simulink library "VariousBlocksLibrary"  (R2015b)
settings: Solver=ode45  StartTime=0.0  StopTime=10.0  RelTol=1e-3
undefined symbols (not defined in the file or in its folder): LopesParams
undefined symbols (not defined in the file): LopesParamsSendDataArrayLen
libraries: simulink x17, dspmtrx3 x9, LopesDevelopmentLibrary x2, LopesLibrary x1, VariousBlocksLibrary x1
(part 1 of 2)
settings Model: xpc_rtwmakecfg_data=_xpcnblib__xpciplib__xpcetherlib__xpcether8255xlib__xpcetherGbElib_  Creator=Administrator  LastModifiedBy=symbitron
settings DataIOCC: SaveFormat=Array  SignalLoggingSaveFormat=ModelDataLogs
settings OptimizationCC: ExpressionDepthLimit=2147483647
settings DebuggingCC: UnderspecifiedInitializationDetection=Classic  MergeDetectMultiDrivingBlocksExec=none  SolverPrmCheckMsg=warning  FcnCallInpInsideContextMsg=UseLocalSettings  StateNameClashWarn=warning
settings HardwareCC: ProdBitPerPointer=32  ProdLargestAtomicFloat=None  ProdIntDivRoundTo=Undefined  ProdEndianess=Unspecified  ProdWordSize=32  ProdHWDeviceType=32-bit Generic
settings GRTTargetCC: GeneratePreprocessorConditionals=Disable all  CombineOutputUpdateFcns=off  GRTInterface=on
settings ConfigComp: CovModelRefEnable=Off

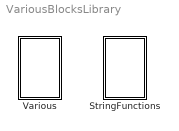
== system VariousBlocksLibrary ==
  StringFunctions : Subsystem
  Various : Subsystem

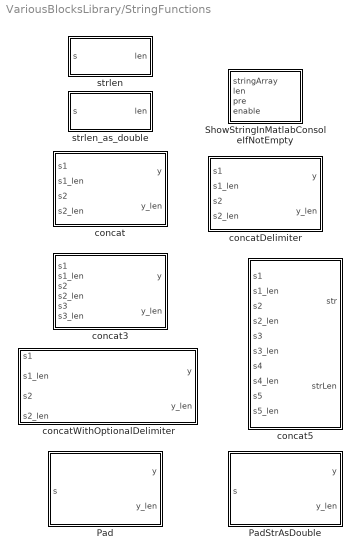
== system VariousBlocksLibrary/StringFunctions ==
  Pad : Subsystem  mask{outArrayLen=100}
      mask prompts: outArrayLen "Size of output array"
  PadStrAsDouble : Subsystem  mask{outArrayLen=LopesParams.exceptionStrArrayLen}
      mask prompts: outArrayLen "Size of output array"
  ShowStringInMatlabConsoleIfNotEmpty : MATLAB Function  TreatAsAtomicUnit=on
  concat : MATLAB Function  TreatAsAtomicUnit=on
  concat3 : MATLAB Function  TreatAsAtomicUnit=on
  concat5 : Subsystem  mask{outStrLen=LopesParamsSendDataArrayLen}
      mask prompts: outStrLen "Length of output array"
  concatDelimiter : MATLAB Function  TreatAsAtomicUnit=on
  concatWithOptionalDelimiter : MATLAB Function  TreatAsAtomicUnit=on
  strlen : MATLAB Function  TreatAsAtomicUnit=on
  strlen_as_double : MATLAB Function  TreatAsAtomicUnit=on

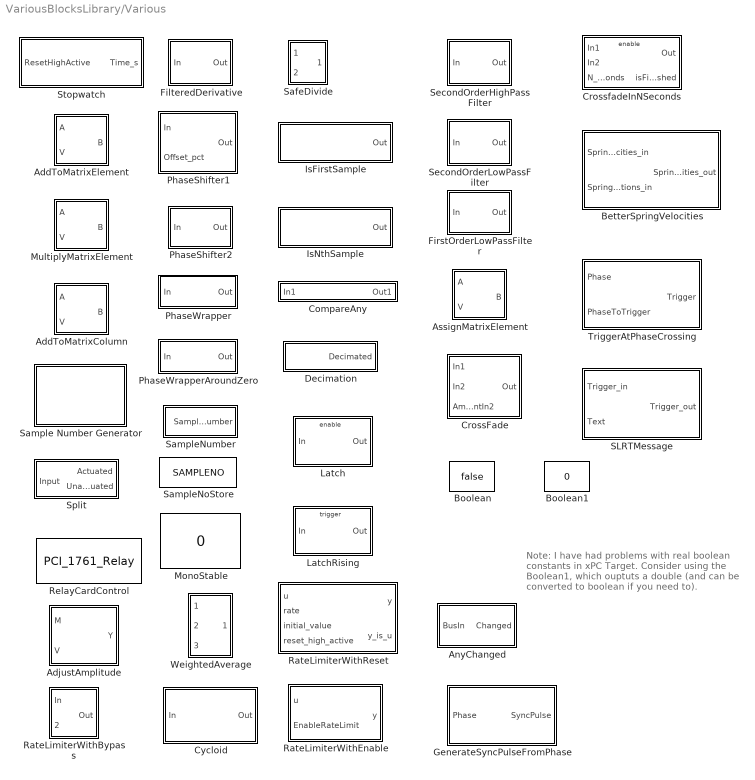
== system VariousBlocksLibrary/Various ==
  note: Note: I have had problems
      | with real boolean constants
      | in xPC Target. Consider
      | using the Boolean1, which ouptuts
      | a double (and can be converted to boolean
      | if you need to).
  AddToMatrixColumn : Subsystem  mask{col=1, minimum=-inf, maximum=inf}
      mask prompts: col "Column (1-based)"
      mask Display:
      | plot([15,10,10,15],[0,0,75,75])
      | plot([70,75,75,70],[0,0,75,75])
      | plot(0,-5)
      | plot(85,85)
      | plot([55,55],[60,70])
      | plot([50,60],[65,65])
      | plot([55,55],[35,45])
      | plot([50,60],[40,40])
      | plot([55,55],[10,20])
      | plot([50,60],[15,15])
  AddToMatrixElement : Subsystem  mask{row=1, col=1, minimum=-inf, maximum=inf}
      mask prompts: row "Row (1-based)"; col "Column (1-based)"
      mask Display:
      | plot([15,10,10,15],[0,0,75,75])
      | plot([70,75,75,70],[0,0,75,75])
      | plot(0,-5)
      | plot(85,85)
      | plot([55,55],[70,60])
      | plot([50,60],[65,65])
  AdjustAmplitude : Subsystem
  AnyChanged : Subsystem
  AssignMatrixElement : Subsystem  mask{row=3, col=2, minimum=-inf, maximum=inf}
      mask prompts: row "Row (1-based)"; col "Column (1-based)"; minimum "Minimum value"; maximum "Maximum value"
      mask Display:
      | plot([15,10,10,15],[0,0,75,75])
      | plot([70,75,75,70],[0,0,75,75])
      | plot(0,-5)
      | plot(85,85)
      | plot([50,60,60,50,50],[60,60,70,70,60])
  BetterSpringVelocities : Subsystem
  Boolean : Constant  Value=false  OutDataTypeStr=boolean
      settings: OpenFcn=|
      | b = get_param(gcb,'value');
      | if (strcmp(b,'true')),
      |   set_param (gcb,'value','false');
      | else
      |   set_param(gcb,'value','true');
      | end;
  Boolean1 : Constant  Value=0  OutDataTypeStr=double
      settings: OpenFcn=|
      | b = get_param(gcb,'value');
      | if (strcmp(b,'1')),
      |   set_param (gcb,'value','0');
      | else
      |   set_param(gcb,'value','1');
      | end;
  CompareAny : Subsystem  mask{values=[3,4]}
      mask Display: disp(['==(',num2strjoin(values,'||'),')'])
  CrossFade : Subsystem
  CrossfadeInNSeconds : Subsystem
  Cycloid : Subsystem
  Decimation : Subsystem  mask{Decimation=1}
      mask prompts: Decimation "Decimation Amount"
      mask TypeOptions Decimation: DecimationAmount/Value
      mask Display: disp(['Decimation: ',num2str(eval(get_param([gcb,'/DecimationAmount'],'Value')))])
  FilteredDerivative : Subsystem  mask{w=10*(2*pi), z=0.7}
      mask prompts: w "Cut off omega [rad/s]"; z "Zeta"
  FirstOrderLowPassFilter : Subsystem  mask{Tau=1}
  GenerateSyncPulseFromPhase : Subsystem
  IsFirstSample : Subsystem  InitFcn=|
      | return; %Disable this becasue it doesnt work!                                                                                                                                                          
      | h = gcb;                                                                                                                                                                                               
      | n = 0; % Number of enable blocks detected upstream                                                                                                                                                     
      | t = []; % type of enable blocks                                                                                                                                                                        
      | while 1,                                                                                                                                                                                               
      |   % Find parent                                                                                                                                                                                        
      |   h = get_param(h,'parent');                                                                                                                                                                           
      |   if (strcmp(h,'')),                                                                                                                                                                                   
      |       % Then we've reached the root                                                                                                                                                                    
      |       break;                                                                                                                                                                                           
      |   end;                                                                                                                                                                                                 
      |   % and check if it has an enable port                                                                                                                                                                 
      |   e = find_system(h,'searchdepth',1, 'BlockType','EnablePort');                                                                                                                                        
      |   if (numel(e)==1),                                                                                                                                                                                    
      |     s = get_param(e{1},'StatesWhenEnabling');                                                                                                                                                          
      |     n=n+1;                                                                                                                                                                                             
      |     if (strcmp(s,'held')),                                                                                                                                                                             
      |         t=[t;'h']; %#ok<AGROW>                                                                                                                                                                         
      |     else                                                                                                                                                                                               
      |         t=[t;'r']; %#ok<AGROW>                                                                                                                                                                         
      |     end;                                                                                                                                                                                               
      |   elseif (numel(e)>1),                                                                                                                                                                                 
      |       error('hun? Multiple enable blocks!')                                                                                                                                                            
      |   end;                                                                                                                                                                                                 
      | end;                                                                                                                                                                                                   
      |                                                                                                                                                                                                        
      | if (n==0),                                                                                                                                                                                             
      |     warning('Warning: %s - The block is not inside an enabled block',gcb)                                                                                                                              
      | elseif (n==1),                                                                                                                                                                                         
      |     if (t(1)=='r')                                                                                                                                                                                     
      |         % This is okay, do nothing                                                                                                                                                                     
      |     else                                                                                                                                                                                               
      |         warning('Warning: %s - This block is inside an enabled block which has its "State when enabling" set to "held". Usually you want it set to "reset" for correct operation.',gcb);               
      |     end;                                                                                                                                                                                               
      | else % n>1                                                                                                                                                                                             
      |     warning('Warning: %s - This block is inside multiple nested enabled blocks. Check which blocks are "held" and which are "reset". You usually want to have at least one "reset" enabled block',gcb);
      | end;
  IsNthSample : Subsystem  InitFcn=|  mask{N=40}
      | return; %Disable this becasue it doesnt work!                                                                                                                                                          
      | h = gcb;                                                                                                                                                                                               
      | n = 0; % Number of enable blocks detected upstream                                                                                                                                                     
      | t = []; % type of enable blocks                                                                                                                                                                        
      | while 1,                                                                                                                                                                                               
      |   % Find parent                                                                                                                                                                                        
      |   h = get_param(h,'parent');                                                                                                                                                                           
      |   if (strcmp(h,'')),                                                                                                                                                                                   
      |       % Then we've reached the root                                                                                                                                                                    
      |       break;                                                                                                                                                                                           
      |   end;                                                                                                                                                                                                 
      |   % and check if it has an enable port                                                                                                                                                                 
      |   e = find_system(h,'searchdepth',1, 'BlockType','EnablePort');                                                                                                                                        
      |   if (numel(e)==1),                                                                                                                                                                                    
      |     s = get_param(e{1},'StatesWhenEnabling');                                                                                                                                                          
      |     n=n+1;                                                                                                                                                                                             
      |     if (strcmp(s,'held')),                                                                                                                                                                             
      |         t=[t;'h']; %#ok<AGROW>                                                                                                                                                                         
      |     else                                                                                                                                                                                               
      |         t=[t;'r']; %#ok<AGROW>                                                                                                                                                                         
      |     end;                                                                                                                                                                                               
      |   elseif (numel(e)>1),                                                                                                                                                                                 
      |       error('hun? Multiple enable blocks!')                                                                                                                                                            
      |   end;                                                                                                                                                                                                 
      | end;                                                                                                                                                                                                   
      |                                                                                                                                                                                                        
      | if (n==0),                                                                                                                                                                                             
      |     warning('Warning: %s - The block is not inside an enabled block',gcb)                                                                                                                              
      | elseif (n==1),                                                                                                                                                                                         
      |     if (t(1)=='r')                                                                                                                                                                                     
      |         % This is okay, do nothing                                                                                                                                                                     
      |     else                                                                                                                                                                                               
      |         warning('Warning: %s - This block is inside an enabled block which has its "State when enabling" set to "held". Usually you want it set to "reset" for correct operation.',gcb);               
      |     end;                                                                                                                                                                                               
      | else % n>1                                                                                                                                                                                             
      |     warning('Warning: %s - This block is inside multiple nested enabled blocks. Check which blocks are "held" and which are "reset". You usually want to have at least one "reset" enabled block',gcb);
      | end;
  Latch : Subsystem  mask{ic=0}
      mask prompts: ic "Initial Condition"
  LatchRising : Subsystem  mask{ic=0}
      mask prompts: ic "Initial Condition"
  MonoStable : Constant  Value=0
      settings: OpenFcn=set_param(gcb,'Value','1');tname = ['toggletimer_' gcb];delete(timerfind('name',tname));t = timer('timerfcn', ['set_param(''',gcb,''',''Value'',''0'')'],'executionmode','singleshot','startdelay',1,'name',tname);start(t);
      mask Display: fprintf('PushToTrigger\n%s',get_param(gcb,'value'))
  MultiplyMatrixElement : Subsystem  mask{row=1, col=1, minimum=-inf, maximum=inf}
      mask prompts: row "Row (1-based)"; col "Column (1-based)"; minimum "Minimum value"; maximum "Maximum value"
      mask Display:
      | plot([15,10,10,15],[0,0,75,75])
      | plot([70,75,75,70],[0,0,75,75])
      | plot(0,-5)
      | plot(85,85)
      | plot([50,60],[70,60])
      | plot([50,60],[60,70])
  PhaseShifter1 : Subsystem
  PhaseShifter2 : Subsystem
  PhaseWrapper : Subsystem
  PhaseWrapperAroundZero : Subsystem
  RateLimiterWithBypass : Subsystem  mask{up=3, down=-3}
      mask prompts: up "Rising slew rate:"; down "Falling slew rate:"
      mask help: If Bypass is nonzero, the rate-limiting functionality is bypassed, and the output is made equal to the input immediately.
  RateLimiterWithEnable : Subsystem  mask{RisingSlewRate=0.5, FallingSlewRate=-0.5}
      mask prompts: RisingSlewRate "Rising Slew Rate:"; FallingSlewRate "Falling Slew Rate:"
  RateLimiterWithReset : Subsystem
  RelayCardControl : S-Function  FunctionName=PCI_1761_Relay  Parameters=baseaddress  SFunctionDeploymentMode=off  EnableBusSupport=off  mask{baseaddress=hex2dec('e000')}
      mask prompts: baseaddress "PCI Base Address (e.g. 0x0300)"
  SLRTMessage : Subsystem
  SafeDivide : Subsystem
      mask Display:
      | port_label('input',1,'X')
      | port_label('input',2,'/')
      | port_label('output',1,'')
  Sample Number Generator : Subsystem
      mask Display: disp('Sample Number\nGenerator')
  SampleNoStore : DataStoreMemory  DataStoreName=SAMPLENO  ReadBeforeWriteMsg=warning  WriteAfterWriteMsg=warning  WriteAfterReadMsg=warning
  SampleNumber : Subsystem
  SecondOrderHighPassFilter : Subsystem  mask{w=10*(2*pi), z=0.7}
      mask prompts: w "Cut off omega [rad/s]"; z "Zeta"
  SecondOrderLowPassFilter : Subsystem  mask{w=10*(2*pi), z=0.7}
      mask prompts: w "Cut off omega [rad/s]"; z "Zeta"
  Split : Subsystem
  Stopwatch : Subsystem
  TriggerAtPhaseCrossing : Subsystem
  WeightedAverage : Subsystem

== system VariousBlocksLibrary/StringFunctions/Pad ==
  s : Inport
  pad : MATLAB Function  TreatAsAtomicUnit=on
  y : Outport
  y_len : Outport  Port=2
  wires:
  pad/1(y) -> y/1
  s/1 -> pad/1(s)
  pad/2(y_len) -> y_len/1

== system VariousBlocksLibrary/StringFunctions/PadStrAsDouble ==
  note: This block pads a string array; the output is as an array of doubles
      | (needed for exception blocks).
  s : Inport
  Data Type Conversion : DataTypeConversion  OutDataTypeStr=double
  pad : MATLAB Function  TreatAsAtomicUnit=on
  y : Outport
  y_len : Outport  Port=2
  wires:
  Data Type Conversion/1 -> y/1
  pad/1(y) -> Data Type Conversion/1
  s/1 -> pad/1(s)
  pad/2(y_len) -> y_len/1

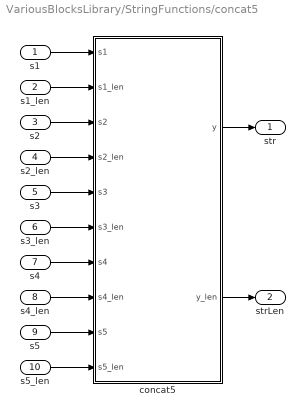
== system VariousBlocksLibrary/StringFunctions/concat5 ==
  s1 : Inport
  s1_len : Inport  Port=2
  s2 : Inport  Port=3
  s2_len : Inport  Port=4
  s3 : Inport  Port=5
  s3_len : Inport  Port=6
  s4 : Inport  Port=7
  s4_len : Inport  Port=8
  s5 : Inport  Port=9
  s5_len : Inport  Port=10
  concat5 : MATLAB Function  TreatAsAtomicUnit=on
  str : Outport
  strLen : Outport  Port=2
  wires:
  s5_len/1 -> concat5/10(s5_len)
  s3_len/1 -> concat5/6(s3_len)
  s3/1 -> concat5/5(s3)
  concat5/1(y) -> str/1
  s1_len/1 -> concat5/2(s1_len)
  s2/1 -> concat5/3(s2)
  s4/1 -> concat5/7(s4)
  s2_len/1 -> concat5/4(s2_len)
  s4_len/1 -> concat5/8(s4_len)
  s5/1 -> concat5/9(s5)
  s1/1 -> concat5/1(s1)
  concat5/2(y_len) -> strLen/1

== system VariousBlocksLibrary/Various/AddToMatrixColumn ==
  A : Inport
  V : Inport  Port=2
  Maximum : Constant  Value=maximum
  Minimum : Constant  Value=minimum
  Overwrite Values : dspmtrx3/Overwrite Values  OverWriteDiag=Submatrix  valFrom2ndIP=Second input port  ConstValue=0  RowSpan=All rows  RowStartMode=Index  RowStartIndex=row  RowEndMode=Last  RowEndIndex=1  ColSpan=One column  ColStartMode=Index  ColStartIndex=col  ColEndMode=Last  ColEndIndex=1  DiagSpan=Range of elements  DiagStartMode=Index  DiagStartIndex=2  DiagEndMode=Index  DiagEndIndex=4
  Saturation Dynamic : simulink/Discontinuities/Saturation Dynamic  OutMin=[]  OutMax=[]  OutDataTypeStr=Inherit: Same as second input  OutDataType=fixdt(1, 16)  OutScaling=2^-10  DoSatur=off
  Submatrix : dspmtrx3/Submatrix  RowSpan=All rows  RowStartMode=Index  RowStartIndex=row  RowEndMode=Index  RowEndIndex=1  ColSpan=One column  ColStartMode=Index  ColStartIndex=col  ColEndMode=Last  ColEndIndex=1
  Sum : Sum  Inputs=|++
  B : Outport
  wires:
  Minimum/1 -> Saturation Dynamic/3
  Maximum/1 -> Saturation Dynamic/1
  Saturation Dynamic/1 -> Overwrite Values/2
  Sum/1 -> Saturation Dynamic/2
  A/1 -> Submatrix/1, Overwrite Values/1
  Overwrite Values/1 -> B/1
  Submatrix/1 -> Sum/1
  V/1 -> Sum/2

== system VariousBlocksLibrary/Various/AddToMatrixElement ==
  A : Inport
  V : Inport  Port=2
  Maximum : Constant  Value=maximum
  Minimum : Constant  Value=minimum
  Overwrite Values : dspmtrx3/Overwrite Values  OverWriteDiag=Submatrix  valFrom2ndIP=Second input port  ConstValue=0  RowSpan=One row  RowStartMode=Index  RowStartIndex=row  RowEndMode=Last  RowEndIndex=1  ColSpan=One column  ColStartMode=Index  ColStartIndex=col  ColEndMode=Last  ColEndIndex=1  DiagSpan=Range of elements  DiagStartMode=Index  DiagStartIndex=2  DiagEndMode=Index  DiagEndIndex=4
  Saturation Dynamic : simulink/Discontinuities/Saturation Dynamic  OutMin=[]  OutMax=[]  OutDataTypeStr=Inherit: Same as second input  OutDataType=fixdt(1, 16)  OutScaling=2^-10  DoSatur=off
  Submatrix : dspmtrx3/Submatrix  RowSpan=One row  RowStartMode=Index  RowStartIndex=row  RowEndMode=Index  RowEndIndex=1  ColSpan=One column  ColStartMode=Index  ColStartIndex=col  ColEndMode=Last  ColEndIndex=1
  Sum : Sum  Inputs=|++
  B : Outport
  wires:
  V/1 -> Sum/2
  Submatrix/1 -> Sum/1
  Overwrite Values/1 -> B/1
  A/1 -> Overwrite Values/1, Submatrix/1
  Sum/1 -> Saturation Dynamic/2
  Saturation Dynamic/1 -> Overwrite Values/2
  Maximum/1 -> Saturation Dynamic/1
  Minimum/1 -> Saturation Dynamic/3

== system VariousBlocksLibrary/Various/AdjustAmplitude ==
  note: This block multiplies all positions, velocities and accelerations by input V;
      | in other words,  it just scales the amplitude of the total curve.
  M : Inport
  V : Inport  Port=2
  Matrix Concatenate : Concatenate  Mode=Multidimensional array  ConcatenateDimension=2
  Product : Product  RndMeth=Zero
  angle_vel_acc : dspmtrx3/Submatrix  RowSpan=All rows  RowStartMode=First  RowStartIndex=1  RowEndMode=Last  RowEndIndex=1  ColSpan=Range of columns  ColStartMode=Index  ColStartIndex=2  ColEndMode=Last  ColEndIndex=1
  times : dspmtrx3/Submatrix  RowSpan=All rows  RowStartMode=First  RowStartIndex=1  RowEndMode=Last  RowEndIndex=1  ColSpan=One column  ColStartMode=First  ColStartIndex=1  ColEndMode=Last  ColEndIndex=1
  Y : Outport
  wires:
  Product/1 -> Matrix Concatenate/2
  times/1 -> Matrix Concatenate/1
  angle_vel_acc/1 -> Product/1
  Matrix Concatenate/1 -> Y/1
  M/1 -> times/1, angle_vel_acc/1
  V/1 -> Product/2

== system VariousBlocksLibrary/Various/AnyChanged ==
  note: Outputs true if any of the bus elements of the inputs changed during this sample.
  BusIn : Inport
  Bus to Vector : BusToVector
  Detect Change : simulink/Logic and Bit Operations/Detect Change  vinit=0  InputProcessing=Inherited  OutDataTypeStr=boolean
  Logical Operator : Logic  Operator=OR  Inputs=1  AllPortsSameDT=off  OutDataTypeStr=boolean
  Changed : Outport
  wires:
  Bus to Vector/1 -> Detect Change/1
  Detect Change/1 -> Logical Operator/1
  BusIn/1 -> Bus to Vector/1
  Logical Operator/1 -> Changed/1

== system VariousBlocksLibrary/Various/AssignMatrixElement ==
  A : Inport
  V : Inport  Port=2
  Maximum : Constant  Value=maximum
  Minimum : Constant  Value=minimum
  Overwrite Values : dspmtrx3/Overwrite Values  OverWriteDiag=Submatrix  valFrom2ndIP=Second input port  ConstValue=0  RowSpan=One row  RowStartMode=Index  RowStartIndex=row  RowEndMode=Last  RowEndIndex=1  ColSpan=One column  ColStartMode=Index  ColStartIndex=col  ColEndMode=Last  ColEndIndex=1  DiagSpan=Range of elements  DiagStartMode=Index  DiagStartIndex=2  DiagEndMode=Index  DiagEndIndex=4
  Saturation Dynamic : simulink/Discontinuities/Saturation Dynamic  OutMin=[]  OutMax=[]  OutDataTypeStr=Inherit: Same as second input  OutDataType=fixdt(1, 16)  OutScaling=2^-10  DoSatur=off
  B : Outport
  wires:
  Minimum/1 -> Saturation Dynamic/3
  Maximum/1 -> Saturation Dynamic/1
  Saturation Dynamic/1 -> Overwrite Values/2
  V/1 -> Saturation Dynamic/2
  Overwrite Values/1 -> B/1
  A/1 -> Overwrite Values/1

== system VariousBlocksLibrary/Various/BetterSpringVelocities ==
  note: If you happen to have the analytical accelerations of the spring positions,
      | you can slightly improve the performance of the system by incorporating them
      | in the velocitiy term. The idea is that the SpringVelocities_in reflect the velocity
      | at (discrete) time t=k, but they will be used throughout the sample, thus  during k<=t<k+1.
      | It would be more accurate to use the velocity halfway that period, i.e. at t=k+0.5. The best
      | estimate of that velocity we can get is by doing first order extrapolation, by using the acceleration.
      | Using Forwarrd Euler, we find v_{k+0.5} = v_k + a_k *0.5*ts, with ts the sample time.
  SpringVelocities_in : Inport
  SpringAccelerations_in : Inport  Port=2
  Add1 : Sum
  EnableAccelerationOptimization : Constant  OutDataTypeStr=double
      settings: OpenFcn=|
      | b = get_param(gcb,'value');
      | if (strcmp(b,'1')),
      |   set_param (gcb,'value','0');
      | else
      |   set_param(gcb,'value','1');
      | end;
  Half : Gain  Gain=0.5
  Product : Product  RndMeth=Zero
  SampleTimeGain : Gain  Gain=LopesParams.ts
  SpringVelocities_out : Outport
  wires:
  EnableAccelerationOptimization/1 -> Product/2
  SampleTimeGain/1 -> Half/1
  SpringAccelerations_in/1 -> SampleTimeGain/1
  Product/1 -> Add1/2
  SpringVelocities_in/1 -> Add1/1
  Add1/1 -> SpringVelocities_out/1
  Half/1 -> Product/1

== system VariousBlocksLibrary/Various/CompareAny ==
  In1 : Inport
  Compare To Constant : simulink/Logic and Bit Operations/Compare To Constant  relop===  const=values  OutDataTypeStr=boolean
  Logical Operator : Logic  Operator=OR  Inputs=1  AllPortsSameDT=off  OutDataTypeStr=boolean
  Out1 : Outport
  wires:
  Logical Operator/1 -> Out1/1
  Compare To Constant/1 -> Logical Operator/1
  In1/1 -> Compare To Constant/1

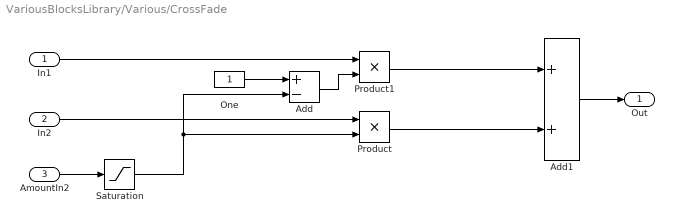
== system VariousBlocksLibrary/Various/CrossFade ==
  In1 : Inport
  In2 : Inport  Port=2
  AmountIn2 : Inport  Port=3
  Add : Sum  Inputs=+-
  Add1 : Sum
  One : Constant
  Product : Product  RndMeth=Zero
  Product1 : Product  RndMeth=Zero
  Saturation : Saturate  UpperLimit=1  LowerLimit=0
  Out : Outport
  wires:
  Add1/1 -> Out/1
  In2/1 -> Product/1
  Product1/1 -> Add1/1
  Product/1 -> Add1/2
  Add/1 -> Product1/2
  Saturation/1 -> Add/2, Product/2
  One/1 -> Add/1
  AmountIn2/1 -> Saturation/1
  In1/1 -> Product1/1

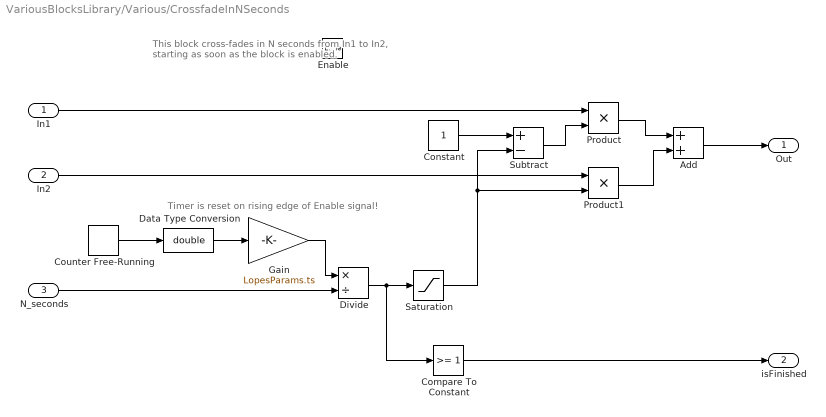
== system VariousBlocksLibrary/Various/CrossfadeInNSeconds ==
  note: This block cross-fades in N seconds from In1 to In2,
      | starting as soon as the block is enabled.
  note: Timer is reset on rising edge of Enable signal!
  In1 : Inport
  In2 : Inport  Port=2
  N_seconds : Inport  Port=3
  Enable : EnablePort  StatesWhenEnabling=reset
  Add : Sum
  Compare To Constant : simulink/Logic and Bit Operations/Compare To Constant  relop=>=  const=1  OutDataTypeStr=boolean
  Constant : Constant
  Counter Free-Running : simulink/Sources/Counter Free-Running  NumBits=32  tsamp=-1
  Data Type Conversion : DataTypeConversion  OutDataTypeStr=double
  Divide : Product  Inputs=*/
  Gain : Gain  Gain=LopesParams.ts
  Product : Product  RndMeth=Zero
  Product1 : Product  RndMeth=Zero
  Saturation : Saturate  UpperLimit=1  LowerLimit=0
  Subtract : Sum  Inputs=+-
  Out : Outport
  isFinished : Outport  Port=2  OutputWhenDisabled=reset  InitialOutput=[0]
  wires:
  Compare To Constant/1 -> isFinished/1
  Divide/1 -> Saturation/1, Compare To Constant/1
  N_seconds/1 -> Divide/2
  Product/1 -> Add/1
  Product1/1 -> Add/2
  Gain/1 -> Divide/1
  Counter Free-Running/1 -> Data Type Conversion/1
  Add/1 -> Out/1
  Data Type Conversion/1 -> Gain/1
  Saturation/1 -> Product1/2, Subtract/2
  In1/1 -> Product/1
  Constant/1 -> Subtract/1
  In2/1 -> Product1/1
  Subtract/1 -> Product/2

== system VariousBlocksLibrary/Various/Cycloid ==
  note: Given a linear input 0<=in<=1, it gives a cycloid output 0<=out<=1.
      | If In is outside the 0..1 range, it is limited to 0 or 1.
  In : Inport
  Gain1 : Gain  Gain=2*pi
  Gain2 : Gain  Gain=1/(2*pi)
  Saturation : Saturate  UpperLimit=1  LowerLimit=0
  Subtract : Sum  Inputs=+-
  Trigonometric Function : Trigonometry
  Out : Outport
  wires:
  Gain2/1 -> Subtract/2
  Trigonometric Function/1 -> Gain2/1
  Saturation/1 -> Subtract/1, Gain1/1
  In/1 -> Saturation/1
  Subtract/1 -> Out/1
  Gain1/1 -> Trigonometric Function/1

== system VariousBlocksLibrary/Various/Decimation ==
  note: This block outputs True  every DecimationAmount'th sample
      | (i.e., if it is 5, it will output True at sample 0, 5, 10, 15, ...).
      | If it is 1, it outputs True all the time.
  Compare To Zero : simulink/Logic and Bit Operations/Compare To Zero  relop===  OutDataTypeStr=boolean  ZeroCross=off
  Counter Free-Running : simulink/Sources/Counter Free-Running  NumBits=32  tsamp=-1
  Data Type Conversion : DataTypeConversion  OutDataTypeStr=double
  DecimationAmount : Constant  Value=Decimation
  Math Function : Math  Operator=mod  SaturateOnIntegerOverflow=on
  Decimated : Outport
  wires:
  Counter Free-Running/1 -> Data Type Conversion/1
  Data Type Conversion/1 -> Math Function/1
  Math Function/1 -> Compare To Zero/1
  DecimationAmount/1 -> Math Function/2
  Compare To Zero/1 -> Decimated/1

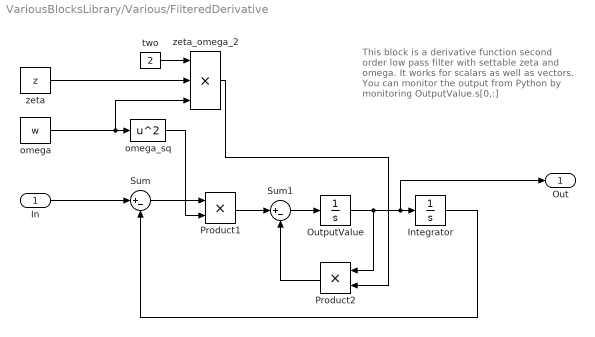
== system VariousBlocksLibrary/Various/FilteredDerivative ==
  note: This block is a derivative function
      | second order low pass filter with
      | settable zeta and omega.
      | It works for scalars as well as vectors.
      |
      | You can monitor the output from Python
      | by monitoring OutputValue.s[0,:]
  In : Inport
  Integrator : Integrator
  OutputValue : Integrator
  Product1 : Product  RndMeth=Zero
  Product2 : Product  RndMeth=Zero
  Sum : Sum  Inputs=|+-
  Sum1 : Sum  Inputs=|+-
  omega : Constant  Value=w
  omega_sq : Math  Operator=square  SaturateOnIntegerOverflow=on
  two : Constant  Value=2
  zeta : Constant  Value=z
  zeta_omega_2 : Product  Inputs=3  RndMeth=Zero
  Out : Outport
  wires:
  Product2/1 -> Sum1/2
  zeta_omega_2/1 -> Product2/2
  Product1/1 -> Sum1/1
  omega_sq/1 -> Product1/2
  zeta/1 -> zeta_omega_2/2
  two/1 -> zeta_omega_2/1
  omega/1 -> omega_sq/1, zeta_omega_2/3
  Sum/1 -> Product1/1
  OutputValue/1 -> Out/1, Integrator/1, Product2/1
  In/1 -> Sum/1
  Sum1/1 -> OutputValue/1
  Integrator/1 -> Sum/2

== system VariousBlocksLibrary/Various/FirstOrderLowPassFilter ==
  In : Inport
  Integrator : Integrator
  OneOverTau : Gain  Gain=1/Tau
  Sum : Sum  Inputs=|+-
  Out : Outport
  wires:
  Sum/1 -> OneOverTau/1
  Integrator/1 -> Sum/2, Out/1
  In/1 -> Sum/1
  OneOverTau/1 -> Integrator/1

== system VariousBlocksLibrary/Various/GenerateSyncPulseFromPhase ==
  note: This block generates a sync pulse.
      | When the phase resets (goes from 100% to 0%),
      | the sync output is set to 1 for a random time (default: between 0.1 and 0.5 s).
      | The fact that the time is random (i.e, not a repeating pattern) allows
      | for absolute syncing of two instances of the sync signal.
  Phase : Inport
  Data Type Conversion : DataTypeConversion  OutDataTypeStr=double
  DetectPhaseSignalReset : Subsystem
  GenerateRandomValue : Subsystem
  MaximumPulseLength_s : Constant  Value=0.5
  MinimumPulseLength_s : Constant  Value=0.1
  Relational Operator : RelationalOperator  Operator=<=  OutDataTypeStr=boolean
  Stopwatch : LopesLibrary/Various/Stopwatch
  SyncPulse : Outport
  wires:
  Data Type Conversion/1 -> SyncPulse/1
  Relational Operator/1 -> Data Type Conversion/1
  Stopwatch/1 -> Relational Operator/1
  GenerateRandomValue/1(Out) -> Relational Operator/2
  MinimumPulseLength_s/1 -> GenerateRandomValue/2(Minimum)
  MaximumPulseLength_s/1 -> GenerateRandomValue/1(Maximum)
  DetectPhaseSignalReset/1(PhaseReset) -> Stopwatch/1, GenerateRandomValue/Trigger
  Phase/1 -> DetectPhaseSignalReset/1(Phase)

== system VariousBlocksLibrary/Various/IsFirstSample ==
  note: This block outputs 1 on the first sample of the enabled block,
      | zero otherwise.
      | Note that it only works if the enable port has
      | "States when enabled" set to "reset"!
  Constant : Constant  Value=0
  Unit Delay : UnitDelay  InitialCondition=1  SampleTime=-1
  Out : Outport
  wires:
  Unit Delay/1 -> Out/1
  Constant/1 -> Unit Delay/1

== system VariousBlocksLibrary/Various/IsNthSample ==
  note: This block outputs 1 on the Nth sample of the enabled block,
      | zero otherwise. Note that this is 0-based (e.g., N=3 is the fourth
      | sample). Note that it only works if the enable port has
      | "States when enabled" set to "reset"!
  Counter Free-Running : simulink/Sources/Counter Free-Running  NumBits=32  tsamp=-1
  N : Constant  Value=N
  Relational Operator : RelationalOperator  Operator===  OutDataTypeStr=boolean
  Out : Outport
  wires:
  N/1 -> Relational Operator/2
  Counter Free-Running/1 -> Relational Operator/1
  Relational Operator/1 -> Out/1

== system VariousBlocksLibrary/Various/Latch ==
  note: Enable == HIGH: OUtput follows input
      | Enable == LOW: Output does not change anymore.
  In : Inport
  Enable : EnablePort
  Out : Outport  InitialOutput=ic
  wires:
  In/1 -> Out/1

== system VariousBlocksLibrary/Various/LatchRising ==
  note: Enable == HIGH: OUtput follows input
      | Enable == LOW: Output does not change anymore.
  In : Inport
  Trigger : TriggerPort  PortDimensions=1
  Out : Outport  InitialOutput=ic
  wires:
  In/1 -> Out/1

== system VariousBlocksLibrary/Various/MultiplyMatrixElement ==
  A : Inport
  V : Inport  Port=2
  Maximum : Constant  Value=maximum
  Minimum : Constant  Value=minimum
  Overwrite Values : dspmtrx3/Overwrite Values  OverWriteDiag=Submatrix  valFrom2ndIP=Second input port  ConstValue=0  RowSpan=One row  RowStartMode=Index  RowStartIndex=row  RowEndMode=Last  RowEndIndex=1  ColSpan=One column  ColStartMode=Index  ColStartIndex=col  ColEndMode=Last  ColEndIndex=1  DiagSpan=Range of elements  DiagStartMode=Index  DiagStartIndex=2  DiagEndMode=Index  DiagEndIndex=4
  Product : Product  RndMeth=Zero
  Saturation Dynamic : simulink/Discontinuities/Saturation Dynamic  OutMin=[]  OutMax=[]  OutDataTypeStr=Inherit: Same as second input  OutDataType=fixdt(1, 16)  OutScaling=2^-10  DoSatur=off
  Submatrix : dspmtrx3/Submatrix  RowSpan=One row  RowStartMode=Index  RowStartIndex=row  RowEndMode=Index  RowEndIndex=1  ColSpan=One column  ColStartMode=Index  ColStartIndex=col  ColEndMode=Last  ColEndIndex=1
  B : Outport
  wires:
  Minimum/1 -> Saturation Dynamic/3
  Maximum/1 -> Saturation Dynamic/1
  Saturation Dynamic/1 -> Overwrite Values/2
  Product/1 -> Saturation Dynamic/2
  V/1 -> Product/2
  Submatrix/1 -> Product/1
  Overwrite Values/1 -> B/1
  A/1 -> Overwrite Values/1, Submatrix/1

== system VariousBlocksLibrary/Various/PhaseShifter1 ==
  In : Inport
  Offset_pct : Inport  Port=2
  Add : Sum
  Constant1 : Constant  Value=100
  ShiftedPhase : Math  Operator=mod  SaturateOnIntegerOverflow=on
  Out : Outport
  wires:
  Add/1 -> ShiftedPhase/1
  Offset_pct/1 -> Add/2
  In/1 -> Add/1
  ShiftedPhase/1 -> Out/1
  Constant1/1 -> ShiftedPhase/2

== system VariousBlocksLibrary/Various/PhaseShifter2 ==
  note: Shifts the phase by 50%
  In : Inport
  Bias : Bias  Bias=50
  Constant1 : Constant  Value=100
  ShiftedPhase : Math  Operator=mod  SaturateOnIntegerOverflow=on
  Out : Outport
  wires:
  Bias/1 -> ShiftedPhase/1
  In/1 -> Bias/1
  ShiftedPhase/1 -> Out/1
  Constant1/1 -> ShiftedPhase/2

== system VariousBlocksLibrary/Various/PhaseWrapper ==
  note: Wraps the input phase such
      | that the output is always
      | in the range 0<=out<100
      | (even if input is negative).
  In : Inport
  Honderd : Constant  Value=100
  ShiftedPhase1 : Math  Operator=mod  SaturateOnIntegerOverflow=on
  Out : Outport
  wires:
  ShiftedPhase1/1 -> Out/1
  In/1 -> ShiftedPhase1/1
  Honderd/1 -> ShiftedPhase1/2

== system VariousBlocksLibrary/Various/PhaseWrapperAroundZero ==
  note: Wraps the input phase such
      | that the output is always
      | in the range -50<=out<50.
      | This is useful for determining the difference
      | (i.e., distance) between two phase signals
  In : Inport
  Bias : Bias  Bias=50
  Honderd : Constant  Value=100
  ShiftedPhase1 : Math  Operator=mod  SaturateOnIntegerOverflow=on
  WrappedOutput : Bias  Bias=-50
  Out : Outport
  wires:
  Honderd/1 -> ShiftedPhase1/2
  In/1 -> Bias/1
  ShiftedPhase1/1 -> WrappedOutput/1
  WrappedOutput/1 -> Out/1
  Bias/1 -> ShiftedPhase1/1

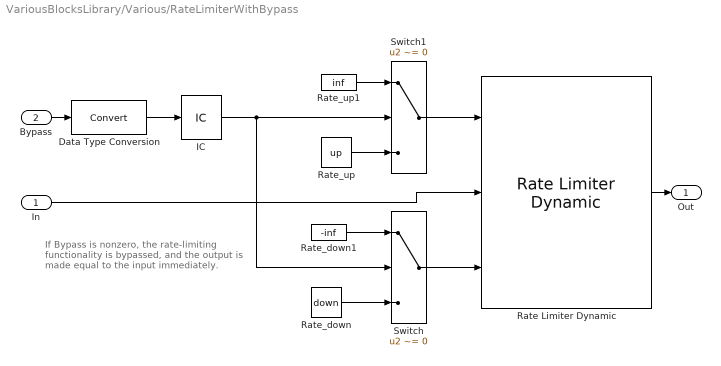
== system VariousBlocksLibrary/Various/RateLimiterWithBypass ==
  note: If Bypass is nonzero, the rate-limiting functionality is bypassed, and the output is made equal to the input immediately.
  In : Inport
  Bypass : Inport  Port=2
  Data Type Conversion : DataTypeConversion
  IC : InitialCondition
  Rate Limiter Dynamic : simulink/Discontinuities/Rate Limiter Dynamic
  Rate_down : Constant  Value=down
  Rate_down1 : Constant  Value=-inf
  "Rate_up " : Constant  Value=up
  Rate_up1 : Constant  Value=inf
  Switch : Switch  Criteria=u2 ~= 0
  Switch1 : Switch  Criteria=u2 ~= 0
  Out : Outport
  wires:
  Data Type Conversion/1 -> IC/1
  IC/1 -> Switch1/2, Switch/2
  Rate_up1/1 -> Switch1/1
  "Rate_up "/1 -> Switch1/3
  Switch1/1 -> Rate Limiter Dynamic/1
  Switch/1 -> Rate Limiter Dynamic/3
  Rate_down/1 -> Switch/3
  Rate_down1/1 -> Switch/1
  In/1 -> Rate Limiter Dynamic/2
  Rate Limiter Dynamic/1 -> Out/1
  Bypass/1 -> Data Type Conversion/1

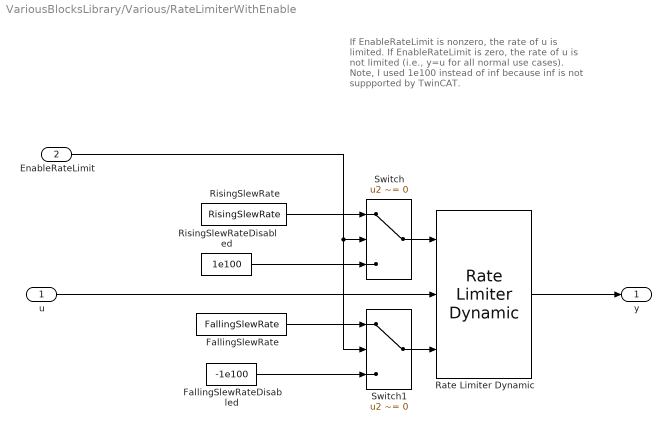
== system VariousBlocksLibrary/Various/RateLimiterWithEnable ==
  note: If EnableRateLimit is nonzero, the rate of u is limited.
      | If EnableRateLimit is zero, the rate of u is not limited (i.e., y=u for all normal use cases).
      | Note, I used 1e100 instead of inf because inf is not suppported by TwinCAT.
  u : Inport
  EnableRateLimit : Inport  Port=2
  FallingSlewRate : Constant  Value=FallingSlewRate
  FallingSlewRateDisabled : Constant  Value=-1e100
  Rate Limiter Dynamic : simulink/Discontinuities/Rate Limiter Dynamic
  RisingSlewRate : Constant  Value=RisingSlewRate
  RisingSlewRateDisabled : Constant  Value=1e100
  Switch : Switch  Criteria=u2 ~= 0
  Switch1 : Switch  Criteria=u2 ~= 0
  y : Outport
  wires:
  FallingSlewRateDisabled/1 -> Switch1/3
  Switch1/1 -> Rate Limiter Dynamic/3
  u/1 -> Rate Limiter Dynamic/2
  Rate Limiter Dynamic/1 -> y/1
  EnableRateLimit/1 -> Switch/2, Switch1/2
  RisingSlewRate/1 -> Switch/1
  RisingSlewRateDisabled/1 -> Switch/3
  Switch/1 -> Rate Limiter Dynamic/1
  FallingSlewRate/1 -> Switch1/1

== system VariousBlocksLibrary/Various/RateLimiterWithReset ==
  u : Inport
  rate : Inport  Port=2
  initial_value : Inport  Port=3
  reset_high_active : Inport  Port=4
  RateLimiterWithReset : MATLAB Function  TreatAsAtomicUnit=on
  y : Outport
  y_is_u : Outport  Port=2
  wires:
  u/1 -> RateLimiterWithReset/1(u)
  RateLimiterWithReset/1(y) -> y/1
  rate/1 -> RateLimiterWithReset/2(rate)
  initial_value/1 -> RateLimiterWithReset/3(initialValue)
  reset_high_active/1 -> RateLimiterWithReset/4(reset_high_active)
  RateLimiterWithReset/2(y_is_u) -> y_is_u/1

== system VariousBlocksLibrary/Various/SLRTMessage ==
  note: This block prints the given text on the SLRT console when Trigger_in is nonzero.
      | It also relays the trigger-in signal. This way, you can put it in front of a StopSimulation
      | block and you're sure that this block is executed first.
      |
      | In its simplest form, the text-input should be a 'constant' block, with as value something like:
      | uint8('This message is printed')
  Trigger_in : Inport
  Text : Inport  Port=2
  Data Type Conversion : DataTypeConversion
  Data Type Conversion1 : DataTypeConversion
  Pad : LopesDevelopmentLibrary/StringFunctions/Pad  outArrayLen=200
  S-Function Builder : S-Function  InitFcn=try, set_param(gcb,'FunctionName','SLRTMessage'), end  FunctionName=SLRTMessage  SFunctionModules=SLRTMessage_wrapper  SFunctionDeploymentMode=off  EnableBusSupport=off  mask(S-Function Builder){}
      mask help: Simulink:masks:SFunctionBuilder_MD
      mask init:
      | val = [[.9  0.75 0.75 1 1 .9 .9 1]',[1 1 0.75 0.75 .9 .9 1 .9]'];try , sys = get_param(gcb,'SfunBuilderFcnName');if isempty(sys), sys = get_param(gcb,'FunctionName'); end,catch, sys = get_param(gcb,'FunctionName'); end
      settings: CopyFcn=set_param(gcbh,'LinkStatus','none')  PreSaveFcn=try, set_param(gcb,'FunctionName','SLRTMessage'), end  OpenFcn=sfunctionwizard(gcbh)
      mask Display: plot(val(:,1),val(:,2)),disp(sys), port_label('input',1,'trigger'), port_label('input',2,'text'), port_label('output',1,'trigger_out')
  Terminator : Terminator
  Trigger_out : Outport
  wires:
  Pad/2 -> Terminator/1
  Data Type Conversion/1 -> S-Function Builder/1
  S-Function Builder/1 -> Data Type Conversion1/1
  Text/1 -> Pad/1
  Pad/1 -> S-Function Builder/2
  Trigger_in/1 -> Data Type Conversion/1
  Data Type Conversion1/1 -> Trigger_out/1

== system VariousBlocksLibrary/Various/SafeDivide ==
  note: This block guarantees division-by-zero-free division.
  Numerator : Inport
  Denominator : Inport  Port=2
  Add : Sum
  Divide : Product  Inputs=*/
  Gain : Gain  Gain=1e-100
  Sign : Signum
  Out : Outport
  wires:
  Gain/1 -> Add/2
  Sign/1 -> Gain/1
  Add/1 -> Divide/2
  Denominator/1 -> Sign/1, Add/1
  Numerator/1 -> Divide/1
  Divide/1 -> Out/1

== system VariousBlocksLibrary/Various/Sample Number Generator ==
  note: Sample Number Generator
      |
      | Put this block once somewhere
      | (preferably in the main window).
      | Then, use the SampleNumber
      | block from the LopesDevelopmentLibrary
      | (in sublibrary Various) to get the
      | sample number.
      | Advantage of using this instead of a
      | free running counter and converter
      | every time you need the sample
      | number:  the sample number is
      | only calculated once, and that disabling blocks
      | does not cause the sample number to freeze.
      |
      | Note: You need to put a DataStore block with
      | identifier SAMPLENO in the main window.
  Counter Free-Running : simulink/Sources/Counter Free-Running  NumBits=32  tsamp=-1
  Data Store Write : DataStoreWrite  DataStoreName=SAMPLENO
  Data Type Conversion : DataTypeConversion  OutDataTypeStr=double
  wires:
  Data Type Conversion/1 -> Data Store Write/1
  Counter Free-Running/1 -> Data Type Conversion/1

== system VariousBlocksLibrary/Various/SampleNumber ==
  note: This block outputs the sample number
      | as a double.
  Data Store Read : DataStoreRead  DataStoreName=SAMPLENO  SampleTime=LopesParams.ts
  SampleNumber : Outport
  wires:
  Data Store Read/1 -> SampleNumber/1

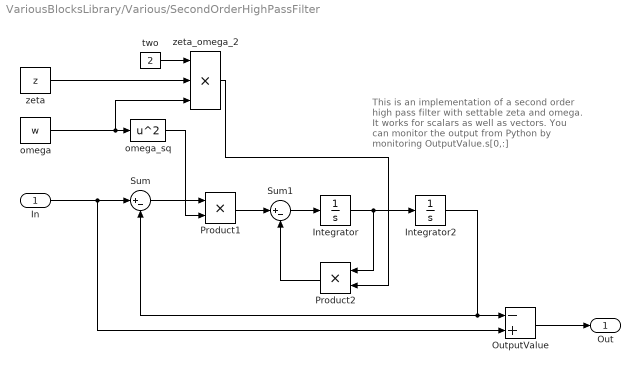
== system VariousBlocksLibrary/Various/SecondOrderHighPassFilter ==
  note: This is an implementation of a
      | second order high pass filter with
      | settable zeta and omega.
      | It works for scalars as well as vectors.
      |
      | You can monitor the output from Python
      | by monitoring OutputValue.s[0,:]
  In : Inport
  Integrator : Integrator
  Integrator2 : Integrator
  OutputValue : Sum  Inputs=-+
  Product1 : Product  RndMeth=Zero
  Product2 : Product  RndMeth=Zero
  Sum : Sum  Inputs=|+-
  Sum1 : Sum  Inputs=|+-
  omega : Constant  Value=w
  omega_sq : Math  Operator=square  SaturateOnIntegerOverflow=on
  two : Constant  Value=2
  zeta : Constant  Value=z
  zeta_omega_2 : Product  Inputs=3  RndMeth=Zero
  Out : Outport
  wires:
  Product2/1 -> Sum1/2
  zeta_omega_2/1 -> Product2/2
  Product1/1 -> Sum1/1
  omega_sq/1 -> Product1/2
  zeta/1 -> zeta_omega_2/2
  two/1 -> zeta_omega_2/1
  omega/1 -> omega_sq/1, zeta_omega_2/3
  Sum/1 -> Product1/1
  Integrator/1 -> Integrator2/1, Product2/1
  In/1 -> OutputValue/2, Sum/1
  Sum1/1 -> Integrator/1
  Integrator2/1 -> OutputValue/1, Sum/2
  OutputValue/1 -> Out/1

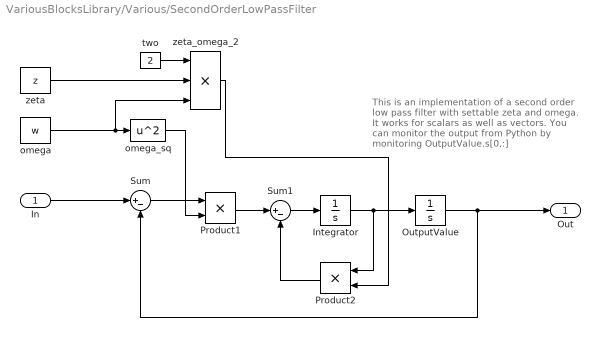
== system VariousBlocksLibrary/Various/SecondOrderLowPassFilter ==
  note: This is an implementation of a
      | second order low pass filter with
      | settable zeta and omega.
      | It works for scalars as well as vectors.
      |
      | You can monitor the output from Python
      | by monitoring OutputValue.s[0,:]
  In : Inport
  Integrator : Integrator
  OutputValue : Integrator
  Product1 : Product  RndMeth=Zero
  Product2 : Product  RndMeth=Zero
  Sum : Sum  Inputs=|+-
  Sum1 : Sum  Inputs=|+-
  omega : Constant  Value=w
  omega_sq : Math  Operator=square  SaturateOnIntegerOverflow=on
  two : Constant  Value=2
  zeta : Constant  Value=z
  zeta_omega_2 : Product  Inputs=3  RndMeth=Zero
  Out : Outport
  wires:
  OutputValue/1 -> Out/1, Sum/2
  Sum1/1 -> Integrator/1
  In/1 -> Sum/1
  Integrator/1 -> Product2/1, OutputValue/1
  Sum/1 -> Product1/1
  omega/1 -> zeta_omega_2/3, omega_sq/1
  two/1 -> zeta_omega_2/1
  zeta/1 -> zeta_omega_2/2
  omega_sq/1 -> Product1/2
  Product1/1 -> Sum1/1
  zeta_omega_2/1 -> Product2/2
  Product2/1 -> Sum1/2

== system VariousBlocksLibrary/Various/Split ==
  note: Thsi block splits up an 11-element vector (containing info
      | of both actuated and unactuated joints) into two
      | parts: the actuated (8-element) and unactauted (3-element) part.
  Input : Inport
  Actuated1 : Selector  InputPortWidth=11  IndexOptions=Index vector (dialog)  Indices=1:8  OutputSizes=1
  Unactuated1 : Selector  InputPortWidth=11  IndexOptions=Index vector (dialog)  Indices=9:11  OutputSizes=1
  Actuated : Outport
  Unactuated : Outport  Port=2
  wires:
  Unactuated1/1 -> Unactuated/1
  Actuated1/1 -> Actuated/1
  Input/1 -> Actuated1/1, Unactuated1/1
